simulink model "k1visetmyt"  (Simulink 8.8)
settings: Solver=ode45  StartTime=0.0  StopTime=10.0  RelTol=1e-3  EnableMultiTasking=on
undefined symbols (not defined in the file): TYPEA_MASTER, TYPEA_TOWER_MASTER
libraries: cdsIPCx x19, cdsCDI64 x4, cdsCDO64 x4, GAS_MODAL_MASTER x4, cdsFilt x4, BIO_CD_ENCODE_MASTER x4, BIO_CD_DECODE_MASTER x4, CHK_DIO x4, cdsEpicsIn x3, TOWER_MASTER x2, VIS_LIB x2, cdsAdcx0 x1
settings Model: SuppressorTable=22 serialization::archive 11 0 3 0 0 0 11 0  Creator=controls  LastModifiedBy=controls
settings DataIOCC: SignalLoggingSaveFormat=Dataset
settings DebuggingCC: UnderspecifiedInitializationDetection=Simplified  MergeDetectMultiDrivingBlocksExec=error  FcnCallInpInsideContextMsg=error  AllowSymbolicDim=off  StateNameClashWarn=none
settings GRTTargetCC: CombineOutputUpdateFcns=on  GRTInterface=off

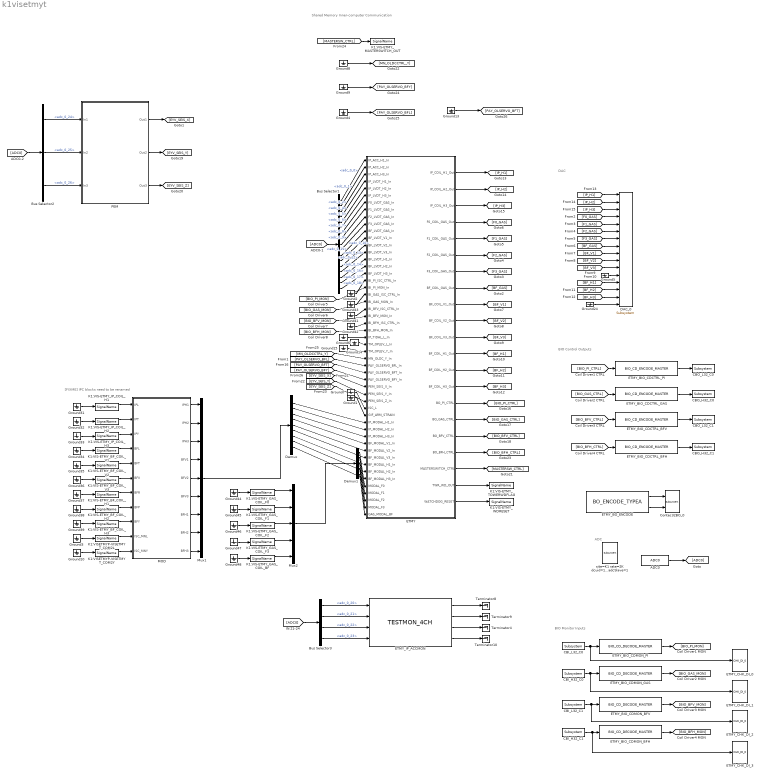
== system k1visetmyt ==
  note: BIO Monitor Inputs
  note: BIO Control Outputs
  note: DAC
  note: ADC
  note: Shared Memory
      | Inner-computer Communication
  note: [FIXME] IPC blocks need to be renamed
  ADC0 : cdsAdcx0/ADC0  Tag=cdsAdc  Description=|
      | type-GSC_16AI64SSA
      | card_num=0
      settings: AttributesFormatString=%<Description>\n%<Tag>
  Bus Selector1 : BusSelector  OutputSignals=adc_0_0,adc_0_1,adc_0_2,adc_0_4,adc_0_5,adc_0_6,adc_0_7,adc_0_8,adc_0_9,adc_0_10,adc_0_11,adc_0_12,adc_0_13,adc_0_14,adc_0_16,adc_0_17,adc_0_18
  Bus Selector2 : BusSelector  OutputSignals=adc_0_24,adc_0_25,adc_0_26
  Bus Selector3 : BusSelector  OutputSignals=adc_0_20,adc_0_21,adc_0_22,adc_0_23
  CBI_H32_C0 : cdsCDI64/Subsystem  Tag=cdsCDI64  Description=card_num=1
      settings: AttributesFormatString=%<Tag>\n%<Description>
  CBI_H32_C1 : cdsCDI64/Subsystem  Tag=cdsCDI64  Description=card_num=3
      settings: AttributesFormatString=%<Tag>\n%<Description>
  CBI_L32_C0 : cdsCDI64/Subsystem  Tag=cdsCDI64  Description=card_num=0
      settings: AttributesFormatString=%<Tag>\n%<Description>
  CBI_L32_C1 : cdsCDI64/Subsystem  Tag=cdsCDI64  Description=card_num=2
      settings: AttributesFormatString=%<Tag>\n%<Description>
  CBO_H32_C0 : cdsCDO64/Subsystem  Tag=cdsCDO64  Description=card_num=1
      settings: AttributesFormatString=%<Tag>\n%<Description>
  CBO_H32_C1 : cdsCDO64/Subsystem  Tag=cdsCDO64  Description=card_num=3
      settings: AttributesFormatString=%<Tag>\n%<Description>
  CBO_L32_C0 : cdsCDO64/Subsystem  Tag=cdsCDO64  Description=card_num=0
      settings: AttributesFormatString=%<Tag>\n%<Description>
  CBO_L32_C1 : cdsCDO64/Subsystem  Tag=cdsCDO64  Description=card_num=2
      settings: AttributesFormatString=%<Tag>\n%<Description>
  Contec32BO_0 : cdsCDO32/Subsystem  Tag=cdsCDO32  Description=Contec32 bit binary output module driver
      settings: AttributesFormatString=%<Tag>
  DAC_0 : dac/Subsystem  Description=|
      | type=GSC_16AO16,
      | card_num=0
      settings: AttributesFormatString=%<Description>
  Demux : Demux  Outputs=9
  Demux1 : Demux  Outputs=5
  ETMY : Subsystem  AncestorBlock=TYPEA_MASTER/TYPEA_TOWER_MASTER
  ETMY_BIO_CDCTRL_BFH : BIO_CD_ENCODE_MASTER/BIO_CD_ENCODE_MASTER
  ETMY_BIO_CDCTRL_BFV : BIO_CD_ENCODE_MASTER/BIO_CD_ENCODE_MASTER
  ETMY_BIO_CDCTRL_GAS : BIO_CD_ENCODE_MASTER/BIO_CD_ENCODE_MASTER
  ETMY_BIO_CDCTRL_PI : BIO_CD_ENCODE_MASTER/BIO_CD_ENCODE_MASTER
  ETMY_BIO_CDMON_BFH : BIO_CD_DECODE_MASTER/BIO_CD_DECODE_MASTER
  ETMY_BIO_CDMON_BFV : BIO_CD_DECODE_MASTER/BIO_CD_DECODE_MASTER
  ETMY_BIO_CDMON_GAS : BIO_CD_DECODE_MASTER/BIO_CD_DECODE_MASTER
  ETMY_BIO_CDMON_PI : BIO_CD_DECODE_MASTER/BIO_CD_DECODE_MASTER
  ETMY_BO_ENCODE : BO_TYPEA_MASTER/BO_ENCODE_TYPEA
  ETMY_CHK_DI_{0..3} (4 alike) : CHK_DIO/CHK_DI_0
  ETMY_IP_ACCMON : TESTMON_4CH_MASTER/TESTMON_4CH
  Ground{1..10,13..15,24,31..39,41..48} (31 alike) : Ground
  K1:VIS-ETMY_BF_COIL_H1 : cdsIPCx/SignalName  Tag=cdsIPCx_SHMEM  Description=Inter-Process Communication via Shared memory.
      settings: AttributesFormatString=%<Tag>
  K1:VIS-ETMY_BF_COIL_H2 : cdsIPCx/SignalName  Tag=cdsIPCx_SHMEM  Description=Inter-Process Communication via Shared memory.
      settings: AttributesFormatString=%<Tag>
  K1:VIS-ETMY_BF_COIL_H3 : cdsIPCx/SignalName  Tag=cdsIPCx_SHMEM  Description=Inter-Process Communication via Shared memory.
      settings: AttributesFormatString=%<Tag>
  K1:VIS-ETMY_BF_COIL_V1 : cdsIPCx/SignalName  Tag=cdsIPCx_SHMEM  Description=Inter-Process Communication via Shared memory.
      settings: AttributesFormatString=%<Tag>
  K1:VIS-ETMY_BF_COIL_V2 : cdsIPCx/SignalName  Tag=cdsIPCx_SHMEM  Description=Inter-Process Communication via Shared memory.
      settings: AttributesFormatString=%<Tag>
  K1:VIS-ETMY_BF_COIL_V3 : cdsIPCx/SignalName  Tag=cdsIPCx_SHMEM  Description=Inter-Process Communication via Shared memory.
      settings: AttributesFormatString=%<Tag>
  K1:VIS-ETMY_GAS_COIL_BF : cdsIPCx/SignalName  Tag=cdsIPCx_SHMEM  Description=Inter-Process Communication via Shared memory.
      settings: AttributesFormatString=%<Tag>
  K1:VIS-ETMY_GAS_COIL_F{0..3} (4 alike) : cdsIPCx/SignalName  Tag=cdsIPCx_SHMEM  Description=Inter-Process Communication via Shared memory.
      settings: AttributesFormatString=%<Tag>
  K1:VIS-ETMY_IP_COIL_H1 : cdsIPCx/SignalName  Tag=cdsIPCx_SHMEM  Description=Inter-Process Communication via Shared memory.
      settings: AttributesFormatString=%<Tag>
  K1:VIS-ETMY_IP_COIL_H2 : cdsIPCx/SignalName  Tag=cdsIPCx_SHMEM  Description=Inter-Process Communication via Shared memory.
      settings: AttributesFormatString=%<Tag>
  K1:VIS-ETMY_IP_COIL_H3 : cdsIPCx/SignalName  Tag=cdsIPCx_SHMEM  Description=Inter-Process Communication via Shared memory.
      settings: AttributesFormatString=%<Tag>
  K1:VIS-ETMY_MASTERSWITCH_OUT : cdsIPCx/SignalName  Tag=cdsIPCx_SHMEM  Description=Inter-Process Communication via Shared memory.
      settings: AttributesFormatString=%<Tag>
  K1:VIS-ETMY_TOWERWDFLAG : cdsIPCx/SignalName  Tag=cdsIPCx_SHMEM  Description=Inter-Process Communication via Shared memory.
      settings: AttributesFormatString=%<Tag>
  K1:VIS-ETMY_WDRESET : cdsIPCx/SignalName  Tag=cdsIPCx_SHMEM  Description=Inter-Process Communication via Shared memory.
      settings: AttributesFormatString=%<Tag>
  K1:VISETMYP-VISETMYT_COM2L : cdsIPCx/SignalName  Tag=cdsIPCx_SHMEM  Description=Inter-Process Communication via Shared memory.
      settings: AttributesFormatString=%<Tag>
  K1:VISETMYP-VISETMYT_COM2Y : cdsIPCx/SignalName  Tag=cdsIPCx_SHMEM  Description=Inter-Process Communication via Shared memory.
      settings: AttributesFormatString=%<Tag>
  MOD : Subsystem  Tag=top_names
  Mux1 : Mux  Inputs=9
  Mux2 : Mux  Inputs=5
  PEM : Subsystem  Tag=top_names
      settings: AttributesFormatString=%<Tag>
  Terminator{4,8..10} (4 alike) : Terminator
  site=K1 rate=2K dcuid=107 host=k1ey1 specific_cpu=2 adcSlave=1 : cdsParameters/Subsystem  Tag=cdsParameters  Description=|
      | Purpose:                                                                                                                                                                                                                                
      | Provide system parameters to the FE code generator to properly configure the generated EPICS names, rep rate of the FE controller, and the Data Acquisition node ID for proper storage of data from this FE controller.                 
      |                                                                                                                                                                                                                                         
      | Useage:                                                                                                                                                                                                                                 
      | The part NAME field is used to identify the FE parameters. It must be of the form:                                                                                                                                                      
      | site=                                                                                                                                                                                                                                   
      | rate=                                                                                                                                                                                                                                   
      | dcuid=                                                                                                                                                                                                                                  
      |                                                                                                                                                                                                                                         
      | Where:                                                                                                                                                                                                                                  
      | site= argument may be H1, H2, L1, M1, G1, either as a single argument or multiple, for example site=H1,H2. These are the only names allowed. These will become the first two characters of all EPICS and signal names (for example G1:).
      |                                                                                                                                                                                                                                         
      | rate= may be 2K, 16K, 32K, or 64K                                                                                                                                                                                                       
      |                                                                                                                                                                                                                                         
      | dcuid= is site specific ie it must be unique at each site.
      settings: AttributesFormatString=%<Tag>
  wires:
  ADC0/1 -> [ADC0]
  ETMY/4(F0_COIL_GAS_Out) -> [F0_GAS]
  ETMY/5(F1_COIL_GAS_Out) -> [F1_GAS]
  ETMY/8(BF_COIL_GAS_Out) -> [BF_GAS]
  ETMY/7(F3_COIL_GAS_Out) -> [F3_GAS]
  ETMY/6(F2_COIL_GAS_Out) -> [F2_GAS]
  ETMY/9(BF_COIL_V1_Out) -> [BF_V1]
  ETMY/10(BF_COIL_V2_Out) -> [BF_V2]
  ETMY/11(BF_COIL_V3_Out) -> [BF_V3]
  ETMY/12(BF_COIL_H1_Out) -> [BF_H1]
  ETMY/13(BF_COIL_H2_Out) -> [BF_H2]
  ETMY/14(BF_COIL_H3_Out) -> [BF_H3]
  [BF_H2] -> DAC_0/14
  [BF_V3] -> DAC_0/11
  [BF_H3] -> DAC_0/15
  [BF_V1] -> DAC_0/9
  [BF_H1] -> DAC_0/13
  [BF_V2] -> DAC_0/10
  ETMY/1(IP_COIL_H1_Out) -> [IP_H1]
  ETMY/2(IP_COIL_H2_Out) -> [IP_H2]
  ETMY/3(IP_COIL_H3_Out) -> [IP_H3]
  CBI_H32_C0/1 -> ETMY_CHK_DI_1/1, ETMY_BIO_CDMON_GAS/1
  CBI_L32_C1/1 -> ETMY_CHK_DI_2/1, ETMY_BIO_CDMON_BFV/1
  CBI_L32_C0/1 -> ETMY_CHK_DI_0/1, ETMY_BIO_CDMON_PI/1
  CBI_H32_C1/1 -> ETMY_CHK_DI_3/1, ETMY_BIO_CDMON_BFH/1
  ETMY_BIO_CDCTRL_BFH/1 -> CBO_H32_C1/1
  ETMY_BIO_CDCTRL_PI/1 -> CBO_L32_C0/1
  ETMY_BIO_CDCTRL_GAS/1 -> CBO_H32_C0/1
  ETMY_BIO_CDCTRL_BFV/1 -> CBO_L32_C1/1
  [BIO_PI_CTRL] -> ETMY_BIO_CDCTRL_PI/1
  [BIO_GAS_CTRL] -> ETMY_BIO_CDCTRL_GAS/1
  [BIO_BFV_CTRL] -> ETMY_BIO_CDCTRL_BFV/1
  ETMY_BIO_CDMON_PI/1 -> [BIO_PI_MON]
  ETMY_BIO_CDMON_GAS/1 -> [BIO_GAS_MON]
  ETMY_BIO_CDMON_BFH/1 -> [BIO_BFH_MON]
  ETMY_BIO_CDMON_BFV/1 -> [BIO_BFV_MON]
  [BIO_BFH_CTRL] -> ETMY_BIO_CDCTRL_BFH/1
  [IP_H1] -> DAC_0/1
  [IP_H2] -> DAC_0/2
  [IP_H3] -> DAC_0/3
  [F0_GAS] -> DAC_0/4
  [F1_GAS] -> DAC_0/5
  [F2_GAS] -> DAC_0/6
  [F3_GAS] -> DAC_0/7
  [BF_GAS] -> DAC_0/8
  [ADC0] -> Bus Selector3/1
  Bus Selector3/2 -> ETMY_IP_ACCMON/2  "<adc_0_21>"
  Bus Selector3/1 -> ETMY_IP_ACCMON/1  "<adc_0_20>"
  Bus Selector3/3 -> ETMY_IP_ACCMON/3  "<adc_0_22>"
  Bus Selector3/4 -> ETMY_IP_ACCMON/4  "<adc_0_23>"
  ETMY_IP_ACCMON/3 -> Terminator4/1
  ETMY_IP_ACCMON/4 -> Terminator10/1
  ETMY_IP_ACCMON/1 -> Terminator8/1
  ETMY_IP_ACCMON/2 -> Terminator9/1
  Ground5/1 -> DAC_0/12
  Ground24/1 -> DAC_0/16
  ETMY/15(BO_PI_CTRL) -> [BIO_PI_CTRL]
  ETMY/16(BO_GAS_CTRL) -> [BIO_GAS_CTRL]
  ETMY/17(BO_BFV_CTRL) -> [BIO_BFV_CTRL]
  ETMY/18(BO_BFH_CTRL) -> [BIO_BFH_CTRL]
  ETMY_BO_ENCODE/1 -> Contec32BO_0/1
  ETMY_BO_ENCODE/2 -> Contec32BO_0/2
  [ADC0] -> Bus Selector1/1
  Bus Selector1/1 -> ETMY/1(IP_ACC_H1_In)  "<adc_0_0>"
  Bus Selector1/2 -> ETMY/2(IP_ACC_H2_In)  "<adc_0_1>"
  Bus Selector1/3 -> ETMY/3(IP_ACC_H3_In)  "<adc_0_2>"
  Bus Selector1/4 -> ETMY/4(IP_LVDT_H1_In)  "<adc_0_4>"
  Bus Selector1/5 -> ETMY/5(IP_LVDT_H2_In)  "<adc_0_5>"
  Bus Selector1/6 -> ETMY/6(IP_LVDT_H3_In)  "<adc_0_6>"
  Bus Selector1/7 -> ETMY/7(F0_LVDT_GAS_In)  "<adc_0_7>"
  Bus Selector1/8 -> ETMY/8(F1_LVDT_GAS_In)  "<adc_0_8>"
  Bus Selector1/9 -> ETMY/9(F2_LVDT_GAS_In)  "<adc_0_9>"
  Bus Selector1/10 -> ETMY/10(F3_LVDT_GAS_In)  "<adc_0_10>"
  Bus Selector1/11 -> ETMY/11(BF_LVDT_GAS_In)  "<adc_0_11>"
  Bus Selector1/12 -> ETMY/12(BF_LVDT_V1_In)  "<adc_0_12>"
  Bus Selector1/13 -> ETMY/13(BF_LVDT_V2_In)  "<adc_0_13>"
  Bus Selector1/14 -> ETMY/14(BF_LVDT_V3_In)  "<adc_0_14>"
  Bus Selector1/15 -> ETMY/15(BF_LVDT_H1_In)  "<adc_0_16>"
  Bus Selector1/16 -> ETMY/16(BF_LVDT_H2_In)  "<adc_0_17>"
  Bus Selector1/17 -> ETMY/17(BF_LVDT_H3_In)  "<adc_0_18>"
  [BIO_PI_MON] -> ETMY/19(BI_PI_MON_In)
  [BIO_GAS_MON] -> ETMY/21(BI_GAS_MON_In)
  [BIO_BFV_MON] -> ETMY/23(BI_BFV_MON_In)
  [BIO_BFH_MON] -> ETMY/25(BI_BFH_MON_In)
  Ground43/1 -> ETMY/20(BI_GAS_ISC_CTRL_In)
  Ground41/1 -> ETMY/22(BI_BFV_ISC_CTRL_In)
  Ground42/1 -> ETMY/24(BI_BFH_ISC_CTRL_In)
  Ground2/1 -> ETMY/18(BI_PI_ISC_CTRL_In)
  Ground8/1 -> [MN_OLDCCTRL_Y]
  Ground9/1 -> [PAY_OLSERVO_BFY]
  Ground4/1 -> [PAY_OLSERVO_BFL]
  Ground13/1 -> [PAY_OLSERVO_BFT]
  Ground14/1 -> ETMY/27(TM_OPLEV_L_In)
  Ground15/1 -> ETMY/28(TM_OPLEV_Y_In)
  ETMY/20(TWR_WD_OUT) -> K1:VIS-ETMY_TOWERWDFLAG/1
  ETMY/21(WATCHDOG_RESET) -> K1:VIS-ETMY_WDRESET/1
  ETMY/19(MASTERSWITCH_CTRL) -> [MASTERSW_CTRL]
  [MASTERSW_CTRL] -> K1:VIS-ETMY_MASTERSWITCH_OUT/1
  Ground1/1 -> ETMY/37(GIF_ARM_STRAIN)
  Ground7/1 -> ETMY/36(ISC_L)
  [PAY_OLSERVO_BFL] -> ETMY/30(PAY_OLSERVO_BFL_In)
  [EYV_SEIS_X] -> ETMY/33(PEM_SEIS_X_In)
  [EYV_SEIS_Y] -> ETMY/34(PEM_SEIS_Y_In)
  [EYV_SEIS_Z] -> ETMY/35(PEM_SEIS_Z_In)
  [MN_OLDCCTRL_Y] -> ETMY/29(MN_OLDC_Y_In)
  [PAY_OLSERVO_BFY] -> ETMY/32(PAY_OLSERVO_BFY_In)
  [PAY_OLSERVO_BFT] -> ETMY/31(PAY_OLSERVO_BFT_In)
  Ground6/1 -> ETMY/26(IP_TIDAL_L_In)
  Mux1/1 -> Demux/1
  Demux/1 -> ETMY/38(IP_MODAL_H1_In)
  Demux/2 -> ETMY/39(IP_MODAL_H2_In)
  Demux/3 -> ETMY/40(IP_MODAL_H3_In)
  Demux/4 -> ETMY/41(BF_MODAL_V1_In)
  Demux/5 -> ETMY/42(BF_MODAL_V2_In)
  Demux/6 -> ETMY/43(BF_MODAL_V3_In)
  Demux/7 -> ETMY/44(BF_MODAL_H1_In)
  Demux/8 -> ETMY/45(BF_MODAL_H2_In)
  Demux/9 -> ETMY/46(BF_MODAL_H3_In)
  [ADC0] -> Bus Selector2/1
  Bus Selector2/1 -> PEM/1(In1)  "<adc_0_24>"
  Bus Selector2/2 -> PEM/2(In2)  "<adc_0_25>"
  Bus Selector2/3 -> PEM/3(In3)  "<adc_0_26>"
  PEM/1(Out1) -> [EYV_SEIS_X]
  PEM/3(Out3) -> [EYV_SEIS_Z]
  PEM/2(Out2) -> [EYV_SEIS_Y]
  Ground31/1 -> K1:VIS-ETMY_IP_COIL_H1/1
  Ground32/1 -> K1:VIS-ETMY_IP_COIL_H2/1
  Ground33/1 -> K1:VIS-ETMY_IP_COIL_H3/1
  Ground34/1 -> K1:VIS-ETMY_BF_COIL_V1/1
  Ground35/1 -> K1:VIS-ETMY_BF_COIL_V2/1
  Ground36/1 -> K1:VIS-ETMY_BF_COIL_V3/1
  Ground37/1 -> K1:VIS-ETMY_BF_COIL_H1/1
  Ground38/1 -> K1:VIS-ETMY_BF_COIL_H2/1
  Ground39/1 -> K1:VIS-ETMY_BF_COIL_H3/1
  K1:VIS-ETMY_IP_COIL_H1/1 -> MOD/1(IPL)
  K1:VIS-ETMY_IP_COIL_H2/1 -> MOD/2(IPT)
  K1:VIS-ETMY_IP_COIL_H3/1 -> MOD/3(IPY)
  K1:VIS-ETMY_BF_COIL_V1/1 -> MOD/4(BFL)
  K1:VIS-ETMY_BF_COIL_V2/1 -> MOD/5(BFT)
  K1:VIS-ETMY_BF_COIL_V3/1 -> MOD/6(BFV)
  K1:VIS-ETMY_BF_COIL_H1/1 -> MOD/7(BFR)
  K1:VIS-ETMY_BF_COIL_H2/1 -> MOD/8(BFP)
  K1:VIS-ETMY_BF_COIL_H3/1 -> MOD/9(BFY)
  MOD/1(IPH1) -> Mux1/1
  MOD/2(IPH2) -> Mux1/2
  MOD/3(IPH3) -> Mux1/3
  MOD/4(BFV1) -> Mux1/4
  MOD/5(BFV2) -> Mux1/5
  MOD/6(BFV3) -> Mux1/6
  MOD/7(BFH1) -> Mux1/7
  MOD/8(BFH2) -> Mux1/8
  MOD/9(BFH3) -> Mux1/9
  K1:VISETMYP-VISETMYT_COM2L/1 -> MOD/10(ISC_MNL)
  K1:VIS-ETMY_GAS_COIL_F0/1 -> Mux2/1
  K1:VIS-ETMY_GAS_COIL_F1/1 -> Mux2/2
  K1:VIS-ETMY_GAS_COIL_F2/1 -> Mux2/3
  K1:VIS-ETMY_GAS_COIL_F3/1 -> Mux2/4
  K1:VIS-ETMY_GAS_COIL_BF/1 -> Mux2/5
  Ground44/1 -> K1:VIS-ETMY_GAS_COIL_F0/1
  Ground45/1 -> K1:VIS-ETMY_GAS_COIL_F1/1
  Ground46/1 -> K1:VIS-ETMY_GAS_COIL_F2/1
  Ground47/1 -> K1:VIS-ETMY_GAS_COIL_F3/1
  Ground48/1 -> K1:VIS-ETMY_GAS_COIL_BF/1
  Mux2/1 -> Demux1/1
  Demux1/1 -> ETMY/47(MODAL_F0)
  Demux1/2 -> ETMY/48(MODAL_F1)
  Demux1/3 -> ETMY/49(MODAL_F2)
  Demux1/4 -> ETMY/50(MODAL_F3)
  Demux1/5 -> ETMY/51(GAS_MODAL_BF)
  K1:VISETMYP-VISETMYT_COM2Y/1 -> MOD/11(ISC_MNY)
  Ground3/1 -> K1:VISETMYP-VISETMYT_COM2L/1
  Ground10/1 -> K1:VISETMYP-VISETMYT_COM2Y/1

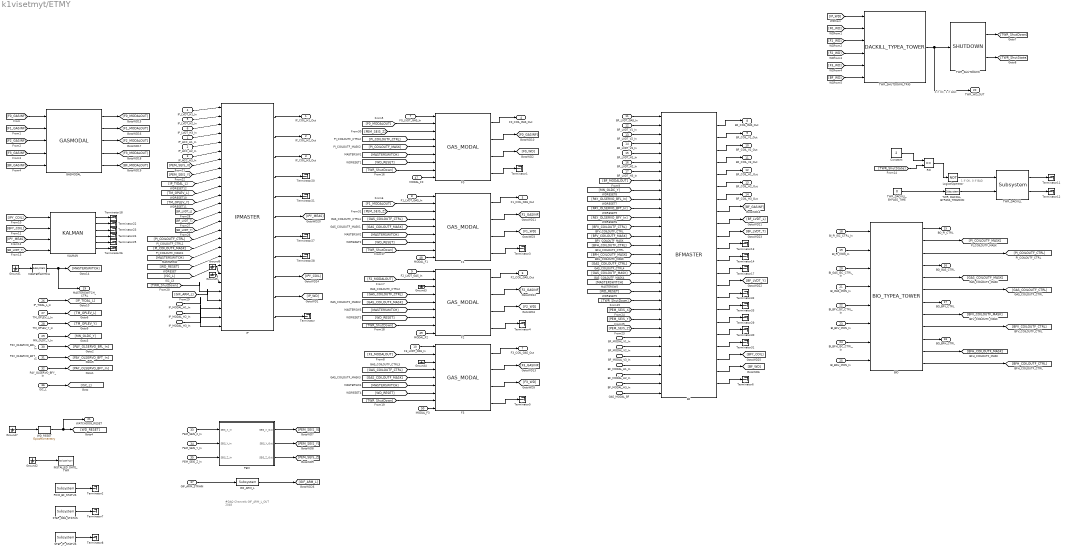
== system k1visetmyt/ETMY ==
  note: #DAQ Channels
      | GIF_ARM_L_OUT 2048
  note: 0 if OK, 1 if BAD
  note: 1 if OK, 0 if BAD
  IP_ACC_H1_In : Inport
  IP_ACC_H2_In : Inport  Port=2
  IP_ACC_H3_In : Inport  Port=3
  IP_LVDT_H1_In : Inport  Port=4
  IP_LVDT_H2_In : Inport  Port=5
  IP_LVDT_H3_In : Inport  Port=6
  F0_LVDT_GAS_In : Inport  Port=7
  F1_LVDT_GAS_In : Inport  Port=8
  F2_LVDT_GAS_In : Inport  Port=9
  F3_LVDT_GAS_In : Inport  Port=10
  BF_LVDT_GAS_In : Inport  Port=11
  BF_LVDT_V1_In : Inport  Port=12
  BF_LVDT_V2_In : Inport  Port=13
  BF_LVDT_V3_In : Inport  Port=14
  BF_LVDT_H1_In : Inport  Port=15
  BF_LVDT_H2_In : Inport  Port=16
  BF_LVDT_H3_In : Inport  Port=17
  BI_PI_ISC_CTRL_In : Inport  Port=18
  BI_PI_MON_In : Inport  Port=19
  BI_GAS_ISC_CTRL_In : Inport  Port=20
  BI_GAS_MON_In : Inport  Port=21
  BI_BFV_ISC_CTRL_In : Inport  Port=22
  BI_BFV_MON_In : Inport  Port=23
  BI_BFH_ISC_CTRL_In : Inport  Port=24
  BI_BFH_MON_In : Inport  Port=25
  IP_TIDAL_L_In : Inport  Port=26
  TM_OPLEV_L_In : Inport  Port=27
  TM_OPLEV_Y_In : Inport  Port=28
  MN_OLDC_Y_In : Inport  Port=29
  PAY_OLSERVO_BFL_In : Inport  Port=30
  PAY_OLSERVO_BFT_In : Inport  Port=31
  PAY_OLSERVO_BFY_In : Inport  Port=32
  PEM_SEIS_X_In : Inport  Port=33
  PEM_SEIS_Y_In : Inport  Port=34
  PEM_SEIS_Z_In : Inport  Port=35
  ISC_L : Inport  Port=36
  GIF_ARM_STRAIN : Inport  Port=37
  IP_MODAL_H1_In : Inport  Port=38
  IP_MODAL_H2_In : Inport  Port=39
  IP_MODAL_H3_In : Inport  Port=40
  BF_MODAL_V1_In : Inport  Port=41
  BF_MODAL_V2_In : Inport  Port=42
  BF_MODAL_V3_In : Inport  Port=43
  BF_MODAL_H1_In : Inport  Port=44
  BF_MODAL_H2_In : Inport  Port=45
  BF_MODAL_H3_In : Inport  Port=46
  MODAL_F0 : Inport  Port=47
  MODAL_F1 : Inport  Port=48
  MODAL_F2 : Inport  Port=49
  MODAL_F3 : Inport  Port=50
  GAS_MODAL_BF : Inport  Port=51
  BF : TOWER_MASTER/BFMASTER
  BIO : BIO_TYPEA_MASTER/BIO_TYPEA_TOWER
  Constant : Constant  Value=2
  F{0..3} (4 alike) : GAS_MODAL_MASTER/GAS_MODAL
  GASMODAL : TYPEA_GAS_MODAL_MASTER/GASMODAL
  GIF_ARM_L : cdsFilt/Subsystem  Tag=cdsFilt  Description=|
      | Purpose:                                                                                                                                                                                                                                  
      | Standard CDS IIR filter module.                                                                                                                                                                                                           
      |                                                                                                                                                                                                                                           
      | Operation:                                                                                                                                                                                                                                
      | Consists of 10 second order section IIR filters, plus a ramped gain stage. In FE code, also provides pre-defined test points and excitation channel inputs. The filter coefficients are defined in the LIGO system using the 'foton' tool.
      |                                                                                                                                                                                                                                           
      | Usage:                                                                                                                                                                                                                                    
      | Name the part with the desired filter module name.
      settings: AttributesFormatString=%<Tag>
  Ground{1..7} (7 alike) : Ground
  INSTALLED_DATE_TWR : cdsEpicsStringIn/EpicsStringIn  Tag=cdsEpicsStringIn  Description=cdsEpicsStringIn
      settings: AttributesFormatString=%<Tag>
  IP : TOWER_MASTER/IPMASTER
  KALMAN : KALMAN_MASTER/KALMAN
  LogicalOperator : Logic  Operator=NOT  AllPortsSameDT=off  OutDataTypeStr=boolean
  MASTERSWITCH : cdsEpicsBinIn/Subsystem  Tag=cdsEpicsBinIn  Description=|
      | Purpose:                                                                            
      | Create an EPICS binary (0 or 1) input channel to the FE realtime controls.          
      |                                                                                     
      | Operation:                                                                          
      | Outputs value from an EPICS ai record. Value is binary input (bi Epics record type).
      |                                                                                     
      | Usage:                                                                              
      | Name the part with the desired EPICS channel name.
      settings: AttributesFormatString=%<Tag>
  PEM : Subsystem
  PICO_BF_STATUS : cdsEpicsIn/Subsystem  Tag=cdsEpicsIn  Description=|
      | Purpose:                                                                              
      | Create an EPICS input channel connection to the FE realtime controls.                 
      |                                                                                       
      | Operation:                                                                            
      | Outputs value from an EPICS ai record. Value is floating point with a precision of 3..
      |                                                                                       
      | Usage:                                                                                
      | Name the part with the desired EPICS channel name.
      settings: AttributesFormatString=%<Tag>
  RO : RelationalOperator  Operator===  OutDataTypeStr=boolean  RndMeth=Nearest
  STEP_GAS_STATUS : cdsEpicsIn/Subsystem  Tag=cdsEpicsIn  Description=|
      | Purpose:                                                                              
      | Create an EPICS input channel connection to the FE realtime controls.                 
      |                                                                                       
      | Operation:                                                                            
      | Outputs value from an EPICS ai record. Value is floating point with a precision of 3..
      |                                                                                       
      | Usage:                                                                                
      | Name the part with the desired EPICS channel name.
      settings: AttributesFormatString=%<Tag>
  STEP_IP_STATUS : cdsEpicsIn/Subsystem  Tag=cdsEpicsIn  Description=|
      | Purpose:                                                                              
      | Create an EPICS input channel connection to the FE realtime controls.                 
      |                                                                                       
      | Operation:                                                                            
      | Outputs value from an EPICS ai record. Value is floating point with a precision of 3..
      |                                                                                       
      | Usage:                                                                                
      | Name the part with the desired EPICS channel name.
      settings: AttributesFormatString=%<Tag>
  TWR_DACKILL : cdsDacKill/Subsystem  Description=cdsDacKill
      settings: AttributesFormatString=%<Description>
  TWR_DACKILL_BYPASS_TIME : Constant  Value=0
  TWR_DACKILL_BYPASS_TIMEMON : cdsEpicsOut/Subsystem  Tag=cdsEpicsOutput  Description=|
      | Purpose:                                          
      | Output a FE signal to an EPICS channel.           
      |                                                   
      | Operation:                                        
      | Takes input value and passes it to EPICS record.  
      |                                                   
      | Usage:                                            
      | Name the part with the desired EPICS rrecord name.
      settings: AttributesFormatString=%<Tag>
  TWR_SHUTDOWN : SHUTDOWN/SHUTDOWN
  TWR_SHUTDOWN_TRIG : VIS_LIB/DACKILL_TYPEA_TOWER
  Terminator{,1..8,11..14,17..18,20..33} (29 alike) : Terminator
  WD_RESET : cdsEpicsMomentary/EpicsMomentary  Tag=cdsEpicsMomentary
      settings: AttributesFormatString=%<Tag>
  IP_COIL_H1_Out : Outport
  IP_COIL_H2_Out : Outport  Port=2
  IP_COIL_H3_Out : Outport  Port=3
  F0_COIL_GAS_Out : Outport  Port=4
  F1_COIL_GAS_Out : Outport  Port=5
  F2_COIL_GAS_Out : Outport  Port=6
  F3_COIL_GAS_Out : Outport  Port=7
  BF_COIL_GAS_Out : Outport  Port=8
  BF_COIL_V1_Out : Outport  Port=9
  BF_COIL_V2_Out : Outport  Port=10
  BF_COIL_V3_Out : Outport  Port=11
  BF_COIL_H1_Out : Outport  Port=12
  BF_COIL_H2_Out : Outport  Port=13
  BF_COIL_H3_Out : Outport  Port=14
  BO_PI_CTRL : Outport  Port=15
  BO_GAS_CTRL : Outport  Port=16
  BO_BFV_CTRL : Outport  Port=17
  BO_BFH_CTRL : Outport  Port=18
  MASTERSWITCH_CTRL : Outport  Port=19
  TWR_WD_OUT : Outport  Port=20
  WATCHDOG_RESET : Outport  Port=21
  wires:
  Ground2/1 -> INSTALLED_DATE_TWR/1
  STEP_IP_STATUS/1 -> Terminator8/1
  STEP_GAS_STATUS/1 -> Terminator7/1
  PICO_BF_STATUS/1 -> Terminator2/1
  IP_TIDAL_L_In/1 -> [IP_TIDAL_L]
  [WD_RESET] -> IP/18
  [PI_COILOUTF_MASK] -> IP/16
  [PI_COILOUTF_CTRL] -> IP/15
  [MASTERSWITCH] -> IP/17
  [ISC_L] -> IP/19
  [TM_OPLEV_Y] -> IP/11
  [TM_OPLEV_L] -> IP/10
  [BF_LVDT_L] -> IP/12
  [BF_LVDT_T] -> IP/13
  [BF_LVDT_Y] -> IP/14
  [IP_TIDAL_L] -> IP/9
  Ground1/1 -> MASTERSWITCH/1
  [PEM_SEIS_Z] -> F0/3
  [PEM_SEIS_Z] -> F1/3
  [TWR_ShutDown] -> F3/8
  [WD_RESET] -> F3/7
  [MASTERSWITCH] -> F3/6
  [GAS_COILOUTF_MASK] -> F3/5
  [GAS_COILOUTF_CTRL] -> F3/4
  Ground4/1 -> F3/3
  [TWR_ShutDown] -> F2/8
  [GAS_COILOUTF_CTRL] -> F2/4
  [WD_RESET] -> F2/7
  [MASTERSWITCH] -> F2/6
  [GAS_COILOUTF_MASK] -> F2/5
  Ground3/1 -> F2/3
  [TWR_ShutDown] -> F1/8
  [WD_RESET] -> F1/7
  [MASTERSWITCH] -> F1/6
  [GAS_COILOUTF_MASK] -> F1/5
  [GAS_COILOUTF_CTRL] -> F1/4
  [TWR_ShutDown] -> F0/8
  [WD_RESET] -> F0/7
  [PI_COILOUTF_MASK] -> F0/5
  [PI_COILOUTF_CTRL] -> F0/4
  [MASTERSWITCH] -> F0/6
  GIF_ARM_STRAIN/1 -> GIF_ARM_L/1
  GIF_ARM_L/1 -> [GIF_ARM_L]
  TM_OPLEV_Y_In/1 -> [TM_OPLEV_Y]
  TM_OPLEV_L_In/1 -> [TM_OPLEV_L]
  PEM_SEIS_Z_In/1 -> PEM/3(SEIS_Z_In)
  PEM_SEIS_X_In/1 -> PEM/1(SEIS_X_In)
  PEM_SEIS_Y_In/1 -> PEM/2(SEIS_Y_In)
  PAY_OLSERVO_BFT_In/1 -> [PAY_OLSERVO_BFT_In]
  PAY_OLSERVO_BFL_In/1 -> [PAY_OLSERVO_BFL_In]
  [BFV_COILOUTF_MASK] -> BF/14
  [GAS_COILOUTF_CTRL] -> BF/17
  [BFV_COILOUTF_CTRL] -> BF/13
  [BFH_COILOUTF_MASK] -> BF/16
  [MASTERSWITCH] -> BF/19
  [PAY_OLSERVO_BFY_In] -> BF/12
  [WD_RESET] -> BF/20
  [TWR_ShutDown] -> BF/21
  [GAS_COILOUTF_MASK] -> BF/18
  [BFH_COILOUTF_CTRL] -> BF/15
  [PEM_SEIS_Z] -> BF/24
  [PAY_OLSERVO_BFT_In] -> BF/11
  [PEM_SEIS_X] -> BF/22
  [PEM_SEIS_Y] -> BF/23
  [PAY_OLSERVO_BFL_In] -> BF/10
  [PEM_SEIS_Y] -> IP/8
  PEM/3(SEIS_Z_Out) -> [PEM_SEIS_Z]
  PEM/2(SEIS_Y_Out) -> [PEM_SEIS_Y]
  [PEM_SEIS_X] -> IP/7
  PEM/1(SEIS_X_Out) -> [PEM_SEIS_X]
  BF/22 -> Terminator6/1
  PAY_OLSERVO_BFY_In/1 -> [PAY_OLSERVO_BFY_In]
  [MN_OLDC_Y] -> BF/9
  IP_LVDT_H2_In/1 -> IP/2
  IP_ACC_H2_In/1 -> IP/5
  IP_LVDT_H1_In/1 -> IP/1
  IP_ACC_H1_In/1 -> IP/4
  IP_LVDT_H3_In/1 -> IP/3
  IP_ACC_H3_In/1 -> IP/6
  IP/1 -> IP_COIL_H1_Out/1
  IP/2 -> IP_COIL_H2_Out/1
  MASTERSWITCH/1 -> [MASTERSWITCH], MASTERSWITCH_CTRL/1
  BF_LVDT_GAS_In/1 -> BF/1
  BF_LVDT_V1_In/1 -> BF/2
  BF_LVDT_V2_In/1 -> BF/3
  BF_LVDT_H2_In/1 -> BF/6
  BF_LVDT_V3_In/1 -> BF/4
  BF_LVDT_H3_In/1 -> BF/7
  BF_LVDT_H1_In/1 -> BF/5
  F1/3 -> [F1_WD]
  F2/3 -> [F2_WD]
  F3/3 -> [F3_WD]
  F1/1 -> F1_COIL_GAS_Out/1
  F2/1 -> F2_COIL_GAS_Out/1
  F3/1 -> F3_COIL_GAS_Out/1
  F1/4 -> Terminator3/1
  F2/4 -> Terminator4/1
  F3/4 -> Terminator5/1
  [IP_WD] -> TWR_SHUTDOWN_TRIG/1
  [F0_WD] -> TWR_SHUTDOWN_TRIG/2
  [F1_WD] -> TWR_SHUTDOWN_TRIG/3
  [F2_WD] -> TWR_SHUTDOWN_TRIG/4
  [F3_WD] -> TWR_SHUTDOWN_TRIG/5
  [BF_WD] -> TWR_SHUTDOWN_TRIG/6
  BI_BFV_ISC_CTRL_In/1 -> BIO/5
  BI_GAS_ISC_CTRL_In/1 -> BIO/3
  BI_BFV_MON_In/1 -> BIO/6
  BI_GAS_MON_In/1 -> BIO/4
  BI_PI_ISC_CTRL_In/1 -> BIO/1
  BI_PI_MON_In/1 -> BIO/2
  BIO/1 -> BO_PI_CTRL/1
  BIO/4 -> BO_GAS_CTRL/1
  BIO/7 -> BO_BFV_CTRL/1
  BIO/2 -> [PI_COILOUTF_MASK]
  BIO/5 -> [GAS_COILOUTF_MASK]
  BIO/8 -> [BFV_COILOUTF_MASK]
  BIO/3 -> [PI_COILOUTF_CTRL]
  BIO/6 -> [GAS_COILOUTF_CTRL]
  BIO/9 -> [BFV_COILOUTF_CTRL]
  BIO/11 -> [BFH_COILOUTF_MASK]
  BIO/12 -> [BFH_COILOUTF_CTRL]
  BIO/10 -> BO_BFH_CTRL/1
  BI_BFH_ISC_CTRL_In/1 -> BIO/7
  BI_BFH_MON_In/1 -> BIO/8
  F0/1 -> F0_COIL_GAS_Out/1
  F0/4 -> Terminator1/1
  F0/3 -> [F0_WD]
  F0_LVDT_GAS_In/1 -> F0/1
  F1_LVDT_GAS_In/1 -> F1/1
  F2_LVDT_GAS_In/1 -> F2/1
  F3_LVDT_GAS_In/1 -> F3/1
  F0/2 -> [F0_GASINF]
  F1/2 -> [F1_GASINF]
  F2/2 -> [F2_GASINF]
  F3/2 -> [F3_GASINF]
  [F2_GASINF] -> GASMODAL/3
  [F3_GASINF] -> GASMODAL/4
  [F1_GASINF] -> GASMODAL/2
  [F0_GASINF] -> GASMODAL/1
  [BF_GASINF] -> GASMODAL/5
  GASMODAL/1 -> [F0_MODALOUT]
  GASMODAL/5 -> [BF_MODALOUT]
  GASMODAL/3 -> [F2_MODALOUT]
  GASMODAL/2 -> [F1_MODALOUT]
  GASMODAL/4 -> [F3_MODALOUT]
  [F0_MODALOUT] -> F0/2
  [F1_MODALOUT] -> F1/2
  [F2_MODALOUT] -> F2/2
  [F3_MODALOUT] -> F3/2
  [BF_MODALOUT] -> BF/8
  BF/1 -> BF_COIL_GAS_Out/1
  BF/2 -> BF_COIL_V1_Out/1
  BF/3 -> BF_COIL_V2_Out/1
  BF/4 -> BF_COIL_V3_Out/1
  BF/5 -> BF_COIL_H1_Out/1
  BF/6 -> BF_COIL_H2_Out/1
  BF/7 -> BF_COIL_H3_Out/1
  BF/8 -> [BF_GASINF]
  BF/9 -> [BF_LVDT_L]
  BF/10 -> [BF_LVDT_T]
  BF/11 -> Terminator13/1
  BF/12 -> Terminator14/1
  BF/13 -> Terminator17/1
  [IPY_COIL] -> KALMAN/1
  [BFY_COIL] -> KALMAN/2
  KALMAN/1 -> Terminator18/1
  KALMAN/2 -> Terminator22/1
  KALMAN/3 -> Terminator23/1
  KALMAN/4 -> Terminator24/1
  KALMAN/5 -> Terminator25/1
  KALMAN/6 -> Terminator26/1
  IP/3 -> IP_COIL_H3_Out/1
  IP/6 -> [IPY_MEAS]
  IP/7 -> Terminator27/1
  IP/8 -> Terminator28/1
  IP/9 -> [IPY_COIL]
  IP/4 -> Terminator20/1
  IP/5 -> Terminator21/1
  IP/10 -> [IP_WD]
  IP/11 -> Terminator/1
  BF/14 -> [BF_LVDT_Y]
  BF/21 -> [BF_WD]
  BF/15 -> Terminator32/1
  BF/16 -> Terminator33/1
  BF/18 -> Terminator30/1
  BF/19 -> Terminator31/1
  BF/17 -> Terminator29/1
  BF/20 -> [BFY_COIL]
  [BF_LVDT_Y] -> KALMAN/4
  [IPY_MEAS] -> KALMAN/3
  MN_OLDC_Y_In/1 -> [MN_OLDC_Y]
  ISC_L/1 -> [ISC_L]
  Ground7/1 -> WD_RESET/1
  WD_RESET/1 -> WATCHDOG_RESET/1, [WD_RESET]
  LogicalOperator/1 -> TWR_DACKILL/1
  TWR_DACKILL_BYPASS_TIMEMON/1 -> TWR_DACKILL/2
  TWR_DACKILL_BYPASS_TIME/1 -> TWR_DACKILL_BYPASS_TIMEMON/1
  TWR_DACKILL/1 -> Terminator11/1
  TWR_DACKILL/2 -> Terminator12/1
  TWR_SHUTDOWN_TRIG/1 -> TWR_WD_OUT/1, TWR_SHUTDOWN/1
  TWR_SHUTDOWN/1 -> [TWR_ShutDown]
  TWR_SHUTDOWN/2 -> [TWR_ShutState]
  Constant/1 -> RO/1
  [TWR_ShutState] -> RO/2
  RO/1 -> LogicalOperator/1
  BF_MODAL_V3_In/1 -> BF/27
  BF_MODAL_V2_In/1 -> BF/26
  BF_MODAL_V1_In/1 -> BF/25
  BF_MODAL_H3_In/1 -> BF/30
  BF_MODAL_H2_In/1 -> BF/29
  BF_MODAL_H1_In/1 -> BF/28
  IP_MODAL_H3_In/1 -> IP/26
  IP_MODAL_H2_In/1 -> IP/25
  IP_MODAL_H1_In/1 -> IP/24
  MODAL_F0/1 -> F0/9
  MODAL_F1/1 -> F1/9
  MODAL_F2/1 -> F2/9
  MODAL_F3/1 -> F3/9
  GAS_MODAL_BF/1 -> BF/31
  [GIF_ARM_L] -> IP/23
  [TWR_ShutDown] -> IP/22
  Ground6/1 -> IP/20
  Ground5/1 -> IP/21

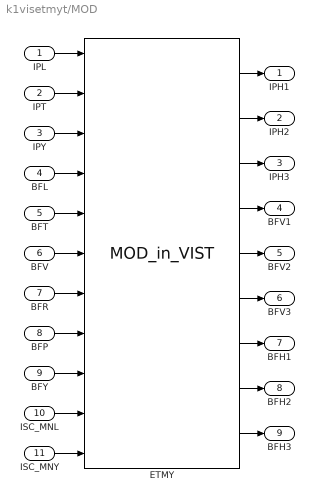
== system k1visetmyt/MOD ==
  IPL : Inport
  IPT : Inport  Port=2
  IPY : Inport  Port=3
  BFL : Inport  Port=4
  BFT : Inport  Port=5
  BFV : Inport  Port=6
  BFR : Inport  Port=7
  BFP : Inport  Port=8
  BFY : Inport  Port=9
  ISC_MNL : Inport  Port=10
  ISC_MNY : Inport  Port=11
  ETMY : VIS_LIB/MODAL/MOD_in_VIST  Tag=top_names
  IPH1 : Outport
  IPH2 : Outport  Port=2
  IPH3 : Outport  Port=3
  BFV1 : Outport  Port=4
  BFV2 : Outport  Port=5
  BFV3 : Outport  Port=6
  BFH1 : Outport  Port=7
  BFH2 : Outport  Port=8
  BFH3 : Outport  Port=9
  wires:
  IPL/1 -> ETMY/1
  IPT/1 -> ETMY/2
  IPY/1 -> ETMY/3
  BFL/1 -> ETMY/4
  BFT/1 -> ETMY/5
  BFV/1 -> ETMY/6
  BFR/1 -> ETMY/7
  BFP/1 -> ETMY/8
  BFY/1 -> ETMY/9
  ETMY/1 -> IPH1/1
  ETMY/2 -> IPH2/1
  ETMY/3 -> IPH3/1
  ETMY/4 -> BFV1/1
  ETMY/5 -> BFV2/1
  ETMY/6 -> BFV3/1
  ETMY/7 -> BFH1/1
  ETMY/8 -> BFH2/1
  ETMY/9 -> BFH3/1
  ISC_MNL/1 -> ETMY/10
  ISC_MNY/1 -> ETMY/11

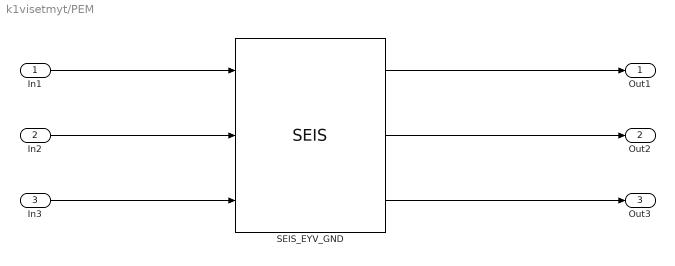
== system k1visetmyt/PEM ==
  In1 : Inport
  In2 : Inport  Port=2
  In3 : Inport  Port=3
  SEIS_EYV_GND : seis/SEIS
  Out1 : Outport
  Out2 : Outport  Port=2
  Out3 : Outport  Port=3
  wires:
  SEIS_EYV_GND/1 -> Out1/1
  SEIS_EYV_GND/2 -> Out2/1
  SEIS_EYV_GND/3 -> Out3/1
  In1/1 -> SEIS_EYV_GND/1
  In2/1 -> SEIS_EYV_GND/2
  In3/1 -> SEIS_EYV_GND/3

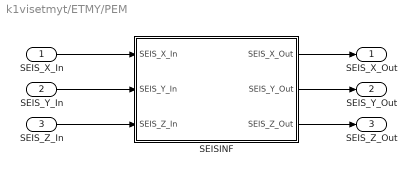
== system k1visetmyt/ETMY/PEM ==
  SEIS_X_In : Inport
  SEIS_Y_In : Inport  Port=2
  SEIS_Z_In : Inport  Port=3
  SEISINF : Subsystem
  SEIS_X_Out : Outport
  SEIS_Y_Out : Outport  Port=2
  SEIS_Z_Out : Outport  Port=3
  wires:
  SEISINF/1(SEIS_X_Out) -> SEIS_X_Out/1
  SEISINF/3(SEIS_Z_Out) -> SEIS_Z_Out/1
  SEISINF/2(SEIS_Y_Out) -> SEIS_Y_Out/1
  SEIS_Z_In/1 -> SEISINF/3(SEIS_Z_In)
  SEIS_Y_In/1 -> SEISINF/2(SEIS_Y_In)
  SEIS_X_In/1 -> SEISINF/1(SEIS_X_In)

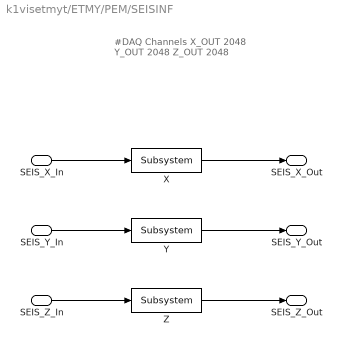
== system k1visetmyt/ETMY/PEM/SEISINF ==
  note: #DAQ Channels
      |
      | X_OUT 2048
      | Y_OUT 2048
      | Z_OUT 2048
  SEIS_X_In : Inport
  SEIS_Y_In : Inport  Port=2
  SEIS_Z_In : Inport  Port=3
  X : cdsFilt/Subsystem  Tag=cdsFilt  Description=|
      | Purpose:                                                                                                                                                                                                                                  
      | Standard CDS IIR filter module.                                                                                                                                                                                                           
      |                                                                                                                                                                                                                                           
      | Operation:                                                                                                                                                                                                                                
      | Consists of 10 second order section IIR filters, plus a ramped gain stage. In FE code, also provides pre-defined test points and excitation channel inputs. The filter coefficients are defined in the LIGO system using the 'foton' tool.
      |                                                                                                                                                                                                                                           
      | Usage:                                                                                                                                                                                                                                    
      | Name the part with the desired filter module name.
      settings: AttributesFormatString=%<Tag>
  Y : cdsFilt/Subsystem  Tag=cdsFilt  Description=|
      | Purpose:                                                                                                                                                                                                                                  
      | Standard CDS IIR filter module.                                                                                                                                                                                                           
      |                                                                                                                                                                                                                                           
      | Operation:                                                                                                                                                                                                                                
      | Consists of 10 second order section IIR filters, plus a ramped gain stage. In FE code, also provides pre-defined test points and excitation channel inputs. The filter coefficients are defined in the LIGO system using the 'foton' tool.
      |                                                                                                                                                                                                                                           
      | Usage:                                                                                                                                                                                                                                    
      | Name the part with the desired filter module name.
      settings: AttributesFormatString=%<Tag>
  Z : cdsFilt/Subsystem  Tag=cdsFilt  Description=|
      | Purpose:                                                                                                                                                                                                                                  
      | Standard CDS IIR filter module.                                                                                                                                                                                                           
      |                                                                                                                                                                                                                                           
      | Operation:                                                                                                                                                                                                                                
      | Consists of 10 second order section IIR filters, plus a ramped gain stage. In FE code, also provides pre-defined test points and excitation channel inputs. The filter coefficients are defined in the LIGO system using the 'foton' tool.
      |                                                                                                                                                                                                                                           
      | Usage:                                                                                                                                                                                                                                    
      | Name the part with the desired filter module name.
      settings: AttributesFormatString=%<Tag>
  SEIS_X_Out : Outport
  SEIS_Y_Out : Outport  Port=2
  SEIS_Z_Out : Outport  Port=3
  wires:
  SEIS_Y_In/1 -> Y/1
  SEIS_X_In/1 -> X/1
  SEIS_Z_In/1 -> Z/1
  X/1 -> SEIS_X_Out/1
  Y/1 -> SEIS_Y_Out/1
  Z/1 -> SEIS_Z_Out/1
